simulink model "simulink51kaskada"  (R2015a)
settings: Solver=FixedStepDiscrete  StartTime=0.0  StopTime=99.0  FixedStep=1  RelTol=1e-3
settings Model: Creator=Bojana Vasic  LastModifiedBy=Bojana Vasic

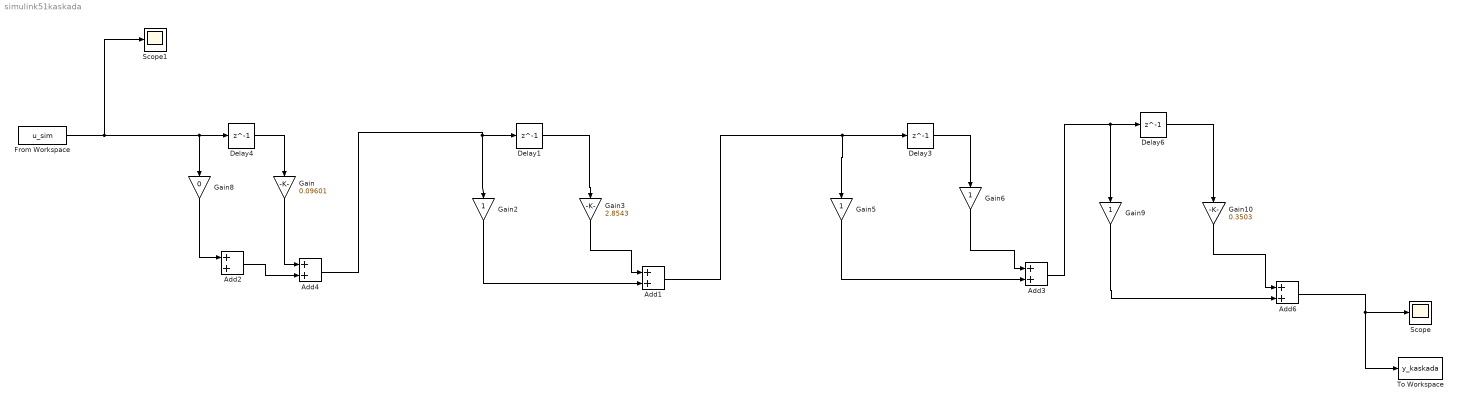
== system simulink51kaskada ==
  Add{1..4,6} (5 alike) : Sum
  Delay{1,3..4,6} (4 alike) : Delay  DelayLength=1
  From Workspace : FromWorkspace  VariableName=u_sim  SampleTime=1
  Gain : Gain  Gain=0.09601
  Gain10 : Gain  Gain=0.3503
  Gain{2,5..6,9} (4 alike) : Gain
  Gain3 : Gain  Gain=2.8543
  Gain8 : Gain  Gain=0
  Scope : Scope
  Scope1 : Scope
  To Workspace : ToWorkspace  VariableName=y_kaskada  SampleTime=-1
      settings: Save2DSignal=2-D array (concatenate along first dimension)
  wires:
  Gain/1 -> Add4/1
  Delay4/1 -> Gain/1
  Delay1/1 -> Gain3/1
  Gain3/1 -> Add1/1
  Gain2/1 -> Add1/2
  Add4/1 -> Delay1/1, Gain2/1
  Delay3/1 -> Gain6/1
  Gain6/1 -> Add3/1
  Gain5/1 -> Add3/2
  Add1/1 -> Gain5/1, Delay3/1
  Delay6/1 -> Gain10/1
  Gain10/1 -> Add6/1
  Gain9/1 -> Add6/2
  Add6/1 -> To Workspace/1, Scope/1
  Add3/1 -> Delay6/1, Gain9/1
  From Workspace/1 -> Delay4/1, Gain8/1, Scope1/1
  Gain8/1 -> Add2/1
  Add2/1 -> Add4/2
